simulink library "lib_plant"  (R2026a)
settings: Solver=VariableStepAuto
undefined symbols (not defined in the file): zs0, zsdot0, zu0, zudot0
settings Model: Creator=alessandro-nardin  LastModifiedBy=alessandro-nardin

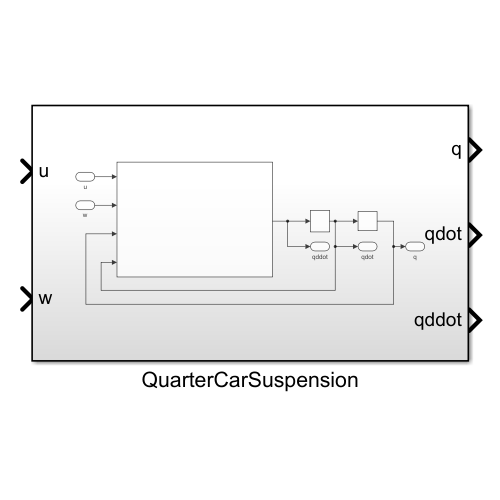
[thumbnail: Simulink's stored preview of the top-level diagram]
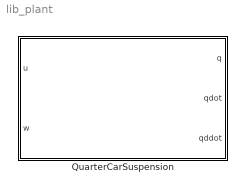
== system lib_plant ==
  QuarterCarSuspension : Subsystem

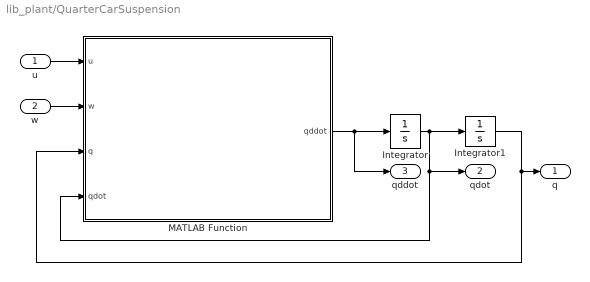
== system lib_plant/QuarterCarSuspension ==
  u : Inport
  w : Inport  Port=2
  Integrator : Integrator  InitialCondition=[ zsdot0; zudot0]
  Integrator1 : Integrator  InitialCondition=[ zs0; zu0 ]
  MATLAB Function : MATLAB Function  TreatAsAtomicUnit=on
  q : Outport
  qdot : Outport  Port=2
  qddot : Outport  Port=3
  wires:
  w/1 -> MATLAB Function/2(w)
  u/1 -> MATLAB Function/1(u)
  Integrator/1 -> qdot/1, MATLAB Function/4(qdot), Integrator1/1
  MATLAB Function/1(qddot) -> qddot/1, Integrator/1
  Integrator1/1 -> MATLAB Function/3(q), q/1

== matlab function lib_plant/QuarterCarSuspension/MATLAB Function ==
  data: u input size=[2 1]; w input size=[2 1]; q input size=[2 1]; qdot input size=[2 1]; qddot output size=[2 1]; plant_param parameter
function qddot = quarter_car_plant_block(u, w, q, qdot, plant_param)
qddot = suspension_dynamics(u, w, q, qdot, plant_param);
